simulink model "LDW"  (R2020b)
settings: Solver=FixedStepAuto  StartTime=0.0  StopTime=Inf  RelTol=1e-3
PostLoadFcn:
  | if any(exist('dsrtsu_mdlpostloadfcn', 'file') ~= 0), dsrtsu_mdlpostloadfcn('Execute', bdroot); end
InitFcn:
  | , if any(exist('dsmpb_private', 'file') ~= 0), dsmpb_private('dsmpb_mdlclblib', 'Init', bdroot); end,
PreSaveFcn:
  | , if any(exist('dsmpb_private', 'file') ~= 0), dsmpb_private('dsmpb_mdlclblib', 'PreSave', bdroot); end,
CloseFcn:
  | , if any(exist('dsmpb_private', 'file') ~= 0), dsmpb_private('dsmpb_mdlclblib', 'Close', bdroot); end,
settings Model: DataDictionary=HWA_DDs.sldd  RTICANMMDATA=struct('GeneralSetupData',struct('modelroot','F:\ADAS_Store\ADAS_Store\Adas\VSM\LSSState\LDW','generalsettings',struct('filesettings',struct('destfolder',struct('Name','RTICANMM_FILES','Check',1),'buildfolder',struct('Name','.','Check',1),'AbsDestfolder',struct('Name','F:\ADAS_Store\ADAS_Store\Adas\VSM\LSSState\LDW\RTICANMM_FILES'),'AbsBuildfolder',struct('Name','F:\ADAS_Store\ADAS_Store\Adas\VSM\LSSState\LDW'))),'options',struct('addpaths',1,'rmpaths',1,'addtrcexclusion',false,'cannavigator',struct('checkmonitoring',0),'show_usrtrc',0,'use_usrtrc',0),'advanced',struct('options',ones(1,100)),'MPSetup',{{}},'RTI',struct('Type','DSRT','Ver','4.2','Date','02-Nov-2019'),'modelname','LDW','block','LDW'))  DSRTSU_INTERNAL_RTIFPGA=150  Creator=GW00199575  LastModifiedBy=GW00199575
settings OptimizationCC: BlockReduction=off  ConditionallyExecuteInputs=off  OptimizeBlockIOStorage=off  BufferReuse=off
settings DebuggingCC: TasksWithSamePriorityMsg=none
settings HardwareCC: ProdBitPerPointer=32  ProdBitPerSizeT=32  ProdBitPerPtrDiffT=32  ProdLargestAtomicInteger=Integer  ProdWordSize=32  ProdHWDeviceType=Custom Processor->Custom
settings ModelReferenceCC: ModelReferenceNumInstancesAllowed=Single
settings SFSimCC: MATLABDynamicMemAlloc=off
settings RTWCC: Description=dSPACE Run-Time Target (for VEOS on Windows and ConfigurationDesk)  SystemTargetFile=dsrt.tlc  GenCodeOnly=on  MakeCommand=make_dsrt  TemplateMakefile=dsrt_default_tmf  RTWVerbose=off
settings CodeAppCC: MaxIdLength=128
settings STFCustomTargetCC: TargetLangStandard=C99 (ISO)  ParMdlRefBuildCompliant=on  ConcurrentExecutionCompliant=off  CPPClassGenCompliant=off  GRTInterface=off  SystemTargetFile=dsrt.tlc
settings GRTTargetCC: CompOptLevelCompliant=off  ConcurrentExecutionCompliant=off  CombineOutputUpdateFcns=off  MatFileLogging=off  CPPClassGenCompliant=off  UseToolchainInfoCompliant=off

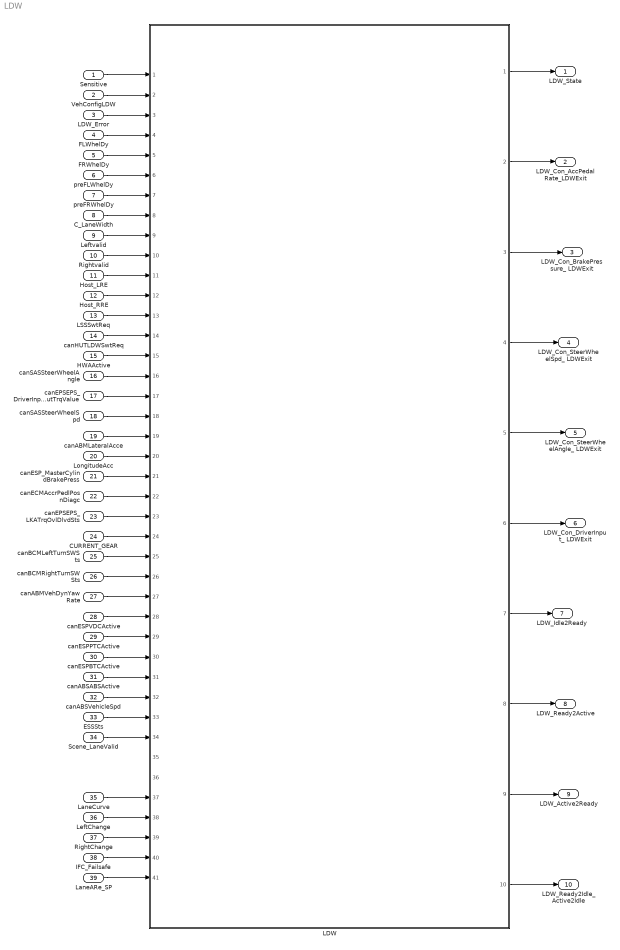
== system LDW ==
  Sensitive : Inport  OutDataTypeStr=uint8
  VehConfigLDW : Inport  Port=2  OutDataTypeStr=uint8
  LDW_Error : Inport  Port=3  OutDataTypeStr=uint8
  FLWhelDy : Inport  Port=4  OutDataTypeStr=single
  FRWhelDy : Inport  Port=5  OutDataTypeStr=single
  preFLWhelDy : Inport  Port=6  OutDataTypeStr=single
  preFRWhelDy : Inport  Port=7  OutDataTypeStr=single
  C_LaneWidth : Inport  Port=8  OutDataTypeStr=single
  Leftvalid : Inport  Port=9  OutDataTypeStr=boolean
  Rightvalid : Inport  Port=10  OutDataTypeStr=boolean
  Host_LRE : Inport  Port=11  OutDataTypeStr=boolean
  Host_RRE : Inport  Port=12  OutDataTypeStr=boolean
  LSSSwtReq : Inport  Port=13  OutDataTypeStr=boolean
  canHUTLDWSwtReq : Inport  Port=14  OutDataTypeStr=boolean
  HWAActive : Inport  Port=15  OutDataTypeStr=boolean
  canSASSteerWheelAngle : Inport  Port=16  OutDataTypeStr=single
  canEPSEPS_DriverInputTrqValue : Inport  Port=17  OutDataTypeStr=single
  canSASSteerWheelSpd : Inport  Port=18  OutDataTypeStr=single
  canABMLateralAcce : Inport  Port=19  OutDataTypeStr=single
  LongitudeAcc : Inport  Port=20  OutDataTypeStr=single
  canESP_MasterCylindBrakePress : Inport  Port=21  OutDataTypeStr=single
  canECMAccrPedlPosnDiagc : Inport  Port=22  OutDataTypeStr=single
  canEPSEPS_LKATrqOvlDlvdSts : Inport  Port=23  OutDataTypeStr=uint8
  CURRENT_GEAR : Inport  Port=24  OutDataTypeStr=uint8
  canBCMLeftTurnSWSts : Inport  Port=25  OutDataTypeStr=boolean
  canBCMRightTurnSWSts : Inport  Port=26  OutDataTypeStr=boolean
  canABMVehDynYawRate : Inport  Port=27  OutDataTypeStr=single
  canESPVDCActive : Inport  Port=28  OutDataTypeStr=boolean
  canESPPTCActive : Inport  Port=29  OutDataTypeStr=boolean
  canESPBTCActive : Inport  Port=30  OutDataTypeStr=boolean
  canABSABSActive : Inport  Port=31  OutDataTypeStr=boolean
  canABSVehicleSpd : Inport  Port=32  OutDataTypeStr=single
  ESSSts : Inport  Port=33  OutDataTypeStr=uint8
  Scene_LaneValid : Inport  Port=34  OutDataTypeStr=single
  LaneCurve : Inport  Port=35  OutDataTypeStr=single
  LeftChange : Inport  Port=36  OutDataTypeStr=boolean
  RightChange : Inport  Port=37  OutDataTypeStr=boolean
  IFC_Failsafe : Inport  Port=38  OutDataTypeStr=double
  LaneARe_SP : Inport  Port=39  OutDataTypeStr=Bus: LaneARe_SP_LDW
  LDW : Subsystem  ReferencedSubsystem=PvtSubSys_VSM_LDW
  LDW_State : Outport
  LDW_Con_AccPedalRate_LDWExit : Outport  Port=2
  LDW_Con_BrakePressure_ LDWExit : Outport  Port=3
  LDW_Con_SteerWheelSpd_ LDWExit : Outport  Port=4
  LDW_Con_SteerWheelAngle_ LDWExit : Outport  Port=5
  LDW_Con_DriverInput_ LDWExit : Outport  Port=6
  LDW_Idle2Ready : Outport  Port=7
  LDW_Ready2Active : Outport  Port=8
  LDW_Active2Ready : Outport  Port=9
  LDW_Ready2Idle_Active2Idle : Outport  Port=10
  wires:
  Sensitive/1 -> LDW/1
  VehConfigLDW/1 -> LDW/2
  LDW_Error/1 -> LDW/3
  FLWhelDy/1 -> LDW/4
  FRWhelDy/1 -> LDW/5
  preFLWhelDy/1 -> LDW/6
  preFRWhelDy/1 -> LDW/7
  C_LaneWidth/1 -> LDW/8
  Leftvalid/1 -> LDW/9
  Rightvalid/1 -> LDW/10
  Host_LRE/1 -> LDW/11
  Host_RRE/1 -> LDW/12
  LSSSwtReq/1 -> LDW/13
  canHUTLDWSwtReq/1 -> LDW/14
  HWAActive/1 -> LDW/15
  canSASSteerWheelAngle/1 -> LDW/16
  canEPSEPS_DriverInputTrqValue/1 -> LDW/17
  canSASSteerWheelSpd/1 -> LDW/18
  canABMLateralAcce/1 -> LDW/19
  LongitudeAcc/1 -> LDW/20
  canESP_MasterCylindBrakePress/1 -> LDW/21
  canECMAccrPedlPosnDiagc/1 -> LDW/22
  canEPSEPS_LKATrqOvlDlvdSts/1 -> LDW/23
  CURRENT_GEAR/1 -> LDW/24
  canBCMLeftTurnSWSts/1 -> LDW/25
  canBCMRightTurnSWSts/1 -> LDW/26
  canABMVehDynYawRate/1 -> LDW/27
  canESPVDCActive/1 -> LDW/28
  canESPPTCActive/1 -> LDW/29
  canESPBTCActive/1 -> LDW/30
  canABSABSActive/1 -> LDW/31
  canABSVehicleSpd/1 -> LDW/32
  ESSSts/1 -> LDW/33
  Scene_LaneValid/1 -> LDW/34
  LDW/7 -> LDW_Idle2Ready/1
  LDW/1 -> LDW_State/1
  LDW/2 -> LDW_Con_AccPedalRate_LDWExit/1
  LDW/8 -> LDW_Ready2Active/1
  LDW/4 -> LDW_Con_SteerWheelSpd_ LDWExit/1
  LDW/9 -> LDW_Active2Ready/1
  LDW/10 -> LDW_Ready2Idle_Active2Idle/1
  LDW/3 -> LDW_Con_BrakePressure_ LDWExit/1
  LDW/5 -> LDW_Con_SteerWheelAngle_ LDWExit/1
  LDW/6 -> LDW_Con_DriverInput_ LDWExit/1
  LaneCurve/1 -> LDW/37
  LeftChange/1 -> LDW/38
  RightChange/1 -> LDW/39
  IFC_Failsafe/1 -> LDW/40
  LaneARe_SP/1 -> LDW/41
